simulink library "navlib1"  (Simulink 3.00)
undefined symbols (not defined in the file): Sloc
libraries: navlib1 x10, simulink3 x4
settings Model: LastModifiedBy=Dutchroll

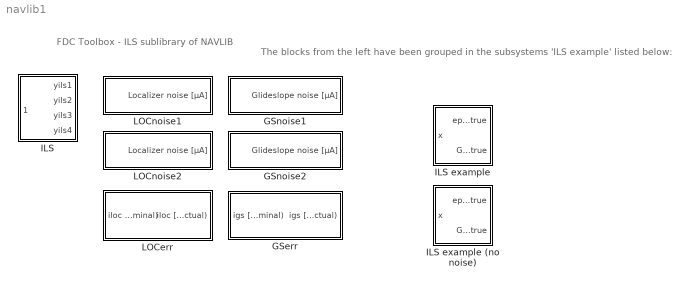
== system navlib1 ==
  note: FDC Toolbox - ILS sublibrary of NAVLIB
  note: The blocks from the left have been
      | grouped in the subsystems
      | 'ILS example' listed below:
  GSerr : Subsystem  mask(GS steady-state errors){cat=2}
      mask prompts: cat "Performance category (1, 2, or 3):"
      mask help: Glideslope steady-state errors
      mask init:
      | gamgs=-abs(@4*pi/180); Sgs=625/abs(gamgs); if cat == 1, D_igs=Sgs*0.075*gamgs; KSgs=1+(@2/100)*0.25; elseif cat == 2, D_igs=Sgs*0.075*gamgs;  KSgs=1+(@2/100)*0.20; else, D_igs=Sgs*0.04*gamgs; KSgs=1+(@2/100)*0.15; end; D_igs=D_igs*@3/100;
      mask Help: eval('browse gserr')
      mask Display: disp('Glideslope steady\nstate errors\nAGARD R-632')
  GSnoise1 : Subsystem  mask(GsNoise1){Lgs=85, sigma_gs=15, V=40}
      mask prompts: Lgs "Scale length Lgs [m]:"; sigma_gs "Standard deviation sigma_gs [µA]:"; V "Approach speed [m/s]:"
      mask help: Glideslope noise (AGARD R-632)
      mask init:
      | K=sigma_gs*sqrt(2*Lgs/V); tau=Lgs/V;
      mask Help: eval('browse gsnoise')
      mask Display: disp('GS noise\nAGARD R-632')
  GSnoise2 : Subsystem
      mask Type: GSNoise NASA-CR2022
      mask Description:
      | Glideslope Noise
      | (NASA-CR2022)
      mask Help: eval('browse gsnoise')
      mask Display: disp('GS noise\nNASA CR-2022')
  ILS : Subsystem  mask(ILS){RWpos=[20000,-100,0]}
      mask prompts: RWpos "Runway heading [deg]:"
      mask help: Approach: ILS
      mask init:
      | psiRW=@1*pi/180; cos_psiRW=cos(psiRW); sin_psiRW=sin(psiRW); xloc=abs(@3); xgs=abs(@4); ygs=-abs(@5); gamgs=-abs(@6)*pi/180; tan_gamgs=tan(gamgs); cos_gamgs=cos(gamgs); Sgs=625/abs(gamgs); if xloc == 0, Sloc = 1; else, Sloc=1.4*xloc; end;
      mask Help: eval('browse ils')
      mask Display: disp('Nominal\nILS\nsignals')
  ILS example : Subsystem
      mask Display: plot(0,0,100,100,[53,23,30,61,53],[45,60,64,49,45],[16,27,32,26],[48,40,43,47],[21,20,24,26,21],[44,55,56,47,44],[20,20,16],[50,50,48],[38,27,26,33],[52,46,48,55],[42,38,27],[50,47,46],[40,44,44,45,45,44,42],[48,44,42,42,44,44,50],[47,45,43],[55,58,58],[54,84,98,90,54],[36,21,56,58,36],[74,68],[34,29],[81,76],[43,38],[87,83],[49,45],[94,89],[57,52],[105,105],[0,0])
  ILS example (no noise) : Subsystem
      mask Display: plot(0,0,100,100,[53,23,30,61,53],[45,60,64,49,45],[16,27,32,26],[48,40,43,47],[21,20,24,26,21],[44,55,56,47,44],[20,20,16],[50,50,48],[38,27,26,33],[52,46,48,55],[42,38,27],[50,47,46],[40,44,44,45,45,44,42],[48,44,42,42,44,44,50],[47,45,43],[55,58,58],[54,84,98,90,54],[36,21,56,58,36],[74,68],[34,29],[81,76],[43,38],[87,83],[49,45],[94,89],[57,52],[105,105],[0,0])
  LOCerr : Subsystem  mask(LOC steady-state errors){cat=2, xloc=2200}
      mask prompts: cat "Performance category (1, 2, or 3):"; xloc "% of max. allowable error in localizer sensitivity:"
      mask help: Localizer steady-state errors
      mask init:
      | Sloc = 1.4*xloc; if cat == 1, D_iloc=Sloc*atan(10.5/xloc); KSloc=1+(@2/100)*0.17; elseif cat == 2, D_iloc=Sloc*atan(7.5/xloc);  KSloc=1+(@2/100)*0.17; else, D_iloc=Sloc*atan(3/xloc); KSloc=1+(@2/100)*0.10; end; D_iloc=D_iloc*@3/100;
      mask Help: eval('browse locerr')
      mask Display: disp('Localizer steady\nstate errors\nAGARD R-632')
  LOCnoise1 : Subsystem  mask(LocNoise1){Lloc=130, sigma_loc=15, V=40}
      mask prompts: Lloc "Scale length Lloc [m]:"; sigma_loc "Standard deviation sigma_loc [µA]:"; V "Approach speed [m/s]:"
      mask help: Localizer noise (AGARD R-632)
      mask init:
      | K=sigma_loc*sqrt(2*Lloc/V); tau=Lloc/V;
      mask Help: eval('browse locnoise')
      mask Display: disp('LOC noise\nAGARD R-632')
  LOCnoise2 : Subsystem
      mask Type: LocNoise 2
      mask Description:
      | Localizer noise
      | (NASA-CR2022)
      mask Help: eval('browse locnoise')
      mask Display: disp('LOC noise\nNASA CR-2022')

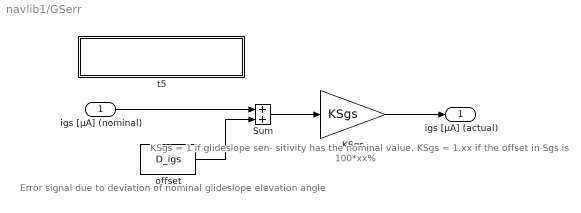
== system navlib1/GSerr ==
  note: KSgs = 1 if glideslope sen-
      | sitivity has the nominal value.
      | KSgs = 1.xx if the offset in
      | Sgs is 100*xx%
  note: Error signal due to deviation
      | of nominal glideslope
      | elevation angle
  igs [µA] (nominal) : Inport  Port=1  PortWidth=-1  SampleTime=-1  DataType=auto
      settings: SignalType=auto
  KSgs : Gain  Gain=KSgs  SaturateOnIntegerOverflow=on
  Sum : Sum  Inputs=++  SaturateOnIntegerOverflow=on
  offset : Constant  Value=D_igs
  t5 : Subsystem
      settings: OpenFcn=browse gserr
      mask Display: disp('Glideslope steady-state errors\nMarc Rauw, April 2003')
  igs [µA] (actual) : Outport  Port=1
  wires:
  offset/1 -> Sum/2
  igs [µA] (nominal)/1 -> Sum/1
  Sum/1 -> KSgs/1
  KSgs/1 -> igs [µA] (actual)/1

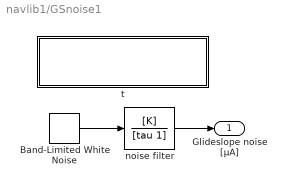
== system navlib1/GSnoise1 ==
  Band-Limited White Noise : simulink3/Sources/Band-Limited White Noise  Cov=[1]  Ts=0.1  seed=[23341]
  noise filter : TransferFcn  Numerator=[K]  Denominator=[tau 1]
  t : Subsystem
      settings: OpenFcn=browse gsnoise
      mask Display: disp('Glideslope noise AGARD R-632\n(constant approach speed)\nMarc Rauw, April 2003')
  Glideslope noise [µA] : Outport  Port=1
  wires:
  Band-Limited White Noise/1 -> noise filter/1
  noise filter/1 -> Glideslope noise [µA]/1

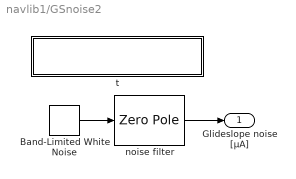
== system navlib1/GSnoise2 ==
  Band-Limited White Noise : simulink3/Sources/Band-Limited White Noise  Cov=[1]  Ts=0.1  seed=[24341]
  noise filter : ZeroPole  Zeros=[]  Poles=[-0.25]  Gain=[3.9875]
  t : Subsystem
      settings: OpenFcn=browse gsnoise
      mask Display: disp('Glideslope noise NASA CR2022\nMarc Rauw, April 2003')
  Glideslope noise [µA] : Outport  Port=1
  wires:
  Band-Limited White Noise/1 -> noise filter/1
  noise filter/1 -> Glideslope noise [µA]/1

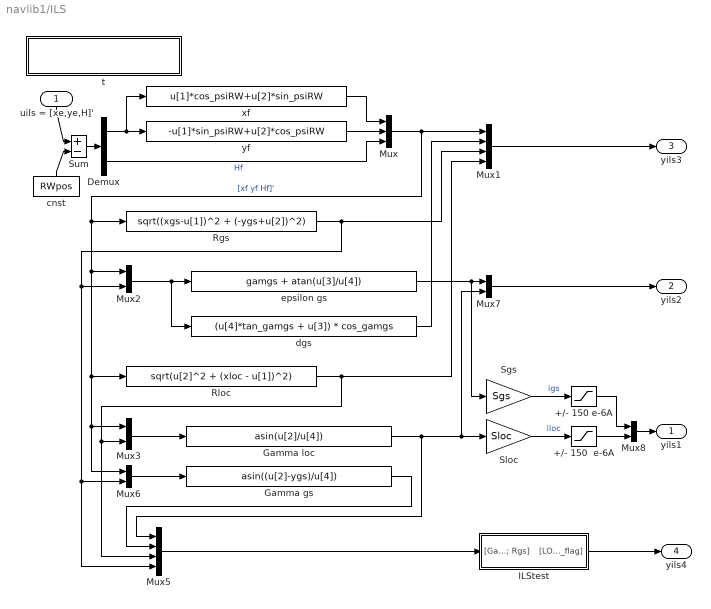
== system navlib1/ILS ==
  uils = [xe,ye,H]' : Inport  Orientation=down  Port=1  PortWidth=-1  SampleTime=-1  DataType=auto
      settings: SignalType=auto
  +/- 150  e-6A : Saturate  UpperLimit=150  LowerLimit=-150
  +/- 150 e-6A : Saturate  UpperLimit=150  LowerLimit=-150
  Demux : Demux  Outputs=[2 1]
  Gamma gs : Fcn  Expr=asin((u[2]-ygs)/u[4])
  Gamma loc : Fcn  Expr=asin(u[2]/u[4])
  ILStest : Subsystem
      mask Type: ILStest
      mask Description: ILS coverage test
      mask Help: eval('browse ilstest')
      mask Display: disp('ILS coverage\ntest (LOC & GS)')
  Mux : Mux  Inputs=3
      settings: DisplayOption=none
  Mux1 : Mux  Inputs=[3 1 1 1]
      settings: DisplayOption=none
  Mux2 : Mux  Inputs=[3 1]
      settings: DisplayOption=none
  Mux3 : Mux  Inputs=[3 1]
      settings: DisplayOption=none
  Mux5 : Mux  Inputs=4
      settings: DisplayOption=none
  Mux6 : Mux  Inputs=[3 1]
      settings: DisplayOption=none
  Mux7 : Mux  Inputs=2
      settings: DisplayOption=none
  Mux8 : Mux  Inputs=2
      settings: DisplayOption=none
  Rgs : Fcn  Expr=sqrt((xgs-u[1])^2 + (-ygs+u[2])^2)
  Rloc : Fcn  Expr=sqrt(u[2]^2 + (xloc - u[1])^2)
  Sgs : Gain  Gain=Sgs  SaturateOnIntegerOverflow=on
  Sloc : Gain  Gain=Sloc  SaturateOnIntegerOverflow=on
  Sum : Sum  Inputs=+-  SaturateOnIntegerOverflow=on
  cnst : Constant  Orientation=up  Value=RWpos
  dgs : Fcn  Expr=(u[4]*tan_gamgs + u[3]) * cos_gamgs
  epsilon gs : Fcn  Expr=gamgs + atan(u[3]/u[4])
  t : Subsystem
      settings: OpenFcn=browse ils
      mask Display: disp('Nominal ILS signals\nM.O. Rauw, February 2004')
  xf : Fcn  Expr=u[1]*cos_psiRW+u[2]*sin_psiRW
  yf : Fcn  Expr=-u[1]*sin_psiRW+u[2]*cos_psiRW
  yils1 : Outport  Port=1
  yils2 : Outport  Port=2
  yils3 : Outport  Port=3
  yils4 : Outport  Port=4
  wires:
  Gamma gs/1 -> Mux5/2
  Mux5/1 -> ILStest/1("[Gamma_loc; Gamma_gs; Rloc; Rgs]")
  ILStest/1("[LOC_flag; GS_flag]") -> yils4/1
  Gamma loc/1 -> Mux5/1, Sloc/1, Mux7/2
  Mux6/1 -> Gamma gs/1
  Mux2/1 -> epsilon gs/1, dgs/1
  Mux1/1 -> yils3/1
  Rloc/1 -> Mux1/4, Mux3/2, Mux5/3
  dgs/1 -> Mux1/2
  Mux3/1 -> Gamma loc/1
  yf/1 -> Mux/2
  xf/1 -> Mux/1
  Sgs/1 -> +/- 150 e-6A/1  "igs"
  Sloc/1 -> +/- 150  e-6A/1  "iloc"
  +/- 150  e-6A/1 -> Mux8/2
  Mux7/1 -> yils2/1
  +/- 150 e-6A/1 -> Mux8/1
  Mux8/1 -> yils1/1
  Rgs/1 -> Mux1/3, Mux2/2, Mux6/2, Mux5/4
  uils = [xe,ye,H]'/1 -> Sum/1
  cnst/1 -> Sum/2
  Demux/2 -> Mux/3  "Hf"
  epsilon gs/1 -> Mux7/1, Sgs/1
  Mux/1 -> Mux2/1, Rloc/1, Mux3/1, Mux6/1, Rgs/1, Mux1/1  "[xf yf Hf]'"
  Sum/1 -> Demux/1
  Demux/1 -> yf/1, xf/1

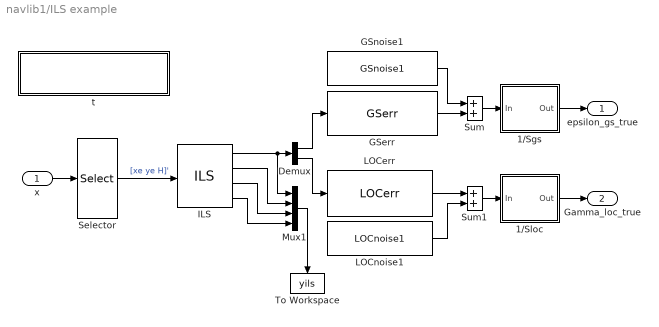
== system navlib1/ILS example ==
  x : Inport  Port=1  PortWidth=-1  SampleTime=-1  DataType=auto
      settings: SignalType=auto
  1/Sgs : Subsystem  mask(1/Sgs){gamgs=-3}
      mask prompts: gamgs "Nominal glideslope angle [deg]:"
      mask help: Multiplication factor 1/Sgs = abs(gamgs)/625, with gamgs the nominal glideslope angle measured in [rad].
      mask init:
      | K = abs(gamgs)*(pi/180)/625;
      mask Help: This block implements a multiplication factor 1/Sgs = abs(gamgs)/625, with gamgs the nominal glideslope angle measured in [rad].
      mask Display: plot([0,100,0,0],[0,50,100,0]);disp('1/Sgs     ');
  1/Sloc : Subsystem  mask(1/Sloc){xloc=2200}
      mask prompts: xloc "Distance from runway threshold to localizer antenna [m]:"
      mask help: Multiplication factor 1/Sloc = 1.40*xloc, with xloc the distance from the runway threshold to the localizer antenna, measured along the runway centerline.
      mask init:
      | K = 1.4*abs(xloc);
      mask Help: This block implements a multiplication factor 1/Sloc = 1.40*xloc, with xloc the distance from the runway threshold to the localizer antenna, measured along the runway centerline.
      mask Display: plot([0,100,0,0],[0,50,100,0]);disp('1/Sloc     ');
  Demux : Demux  Outputs=2
  GSerr : navlib1/GSerr  cat=2  MaskParam2=100  MaskParam3=100  MaskParam4=-3
  GSnoise1 : navlib1/GSnoise1  Lgs=85  sigma_gs=15  V=40
  ILS : navlib1/ILS  RWpos=[20000,-100,0]  MaskParam1=0  MaskParam3=2200  MaskParam4=300  MaskParam5=100  MaskParam6=3
  LOCerr : navlib1/LOCerr  cat=2  xloc=2200  MaskParam2=100  MaskParam3=100
  LOCnoise1 : navlib1/LOCnoise1  Lloc=130  sigma_loc=15  V=40
  Mux1 : Mux  Inputs=[2 2 6 2]
      settings: DisplayOption=none
  Selector : Selector  Elements=[10 11 12]  InputPortWidth=12
  Sum : Sum  Inputs=++  SaturateOnIntegerOverflow=on
  Sum1 : Sum  Inputs=++  SaturateOnIntegerOverflow=on
  To Workspace : ToWorkspace  VariableName=yils  SampleTime=0  SaveFormat=Matrix
      settings: Orientation=down  Buffer=5000
  t : Subsystem
      settings: OpenFcn=browse ilsxmpl
      mask Display: disp('ILS example\nMarc Rauw, January 2005')
  epsilon_gs_true : Outport  Port=1
  Gamma_loc_true : Outport  Port=2
  wires:
  Selector/1 -> ILS/1  "[xe ye H]'"
  Mux1/1 -> To Workspace/1
  Demux/1 -> GSerr/1
  Demux/2 -> LOCerr/1
  ILS/4 -> Mux1/4
  ILS/1 -> Demux/1, Mux1/1
  ILS/3 -> Mux1/3
  ILS/2 -> Mux1/2
  GSerr/1 -> Sum/2
  LOCnoise1/1 -> Sum1/2
  GSnoise1/1 -> Sum/1
  LOCerr/1 -> Sum1/1
  Sum1/1 -> 1/Sloc/1(In)
  Sum/1 -> 1/Sgs/1(In)
  x/1 -> Selector/1
  1/Sgs/1(Out) -> epsilon_gs_true/1
  1/Sloc/1(Out) -> Gamma_loc_true/1

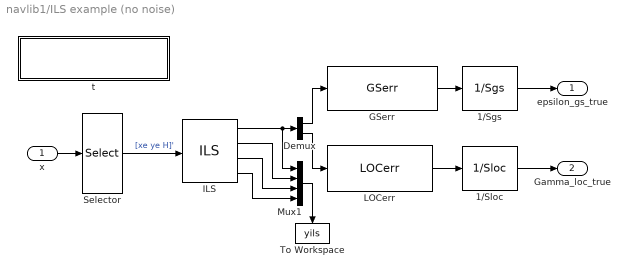
== system navlib1/ILS example (no noise) ==
  x : Inport  Port=1  PortWidth=-1  SampleTime=-1  DataType=auto
      settings: SignalType=auto
  1/Sgs : navlib1/ILS example/1//Sgs  gamgs=-3
  1/Sloc : navlib1/ILS example/1//Sloc  xloc=2200
  Demux : Demux  Outputs=2
  GSerr : navlib1/GSerr  cat=2  MaskParam2=100  MaskParam3=100  MaskParam4=-3
  ILS : navlib1/ILS  RWpos=[20000,-100,0]  MaskParam1=0  MaskParam3=2200  MaskParam4=300  MaskParam5=100  MaskParam6=3
  LOCerr : navlib1/LOCerr  cat=2  xloc=2200  MaskParam2=100  MaskParam3=100
  Mux1 : Mux  Inputs=[2 2 6 2]
      settings: DisplayOption=none
  Selector : Selector  Elements=[10 11 12]  InputPortWidth=12
  To Workspace : ToWorkspace  VariableName=yils  SampleTime=0  SaveFormat=Matrix
      settings: Orientation=down  Buffer=5000
  t : Subsystem
      settings: OpenFcn=browse ilsxmpl
      mask Display: disp('ILS example (no noise)\nMarc Rauw, January 2005')
  epsilon_gs_true : Outport  Port=1
  Gamma_loc_true : Outport  Port=2
  wires:
  Selector/1 -> ILS/1  "[xe ye H]'"
  ILS/2 -> Mux1/2
  ILS/3 -> Mux1/3
  ILS/1 -> Mux1/1, Demux/1
  ILS/4 -> Mux1/4
  Demux/2 -> LOCerr/1
  Demux/1 -> GSerr/1
  Mux1/1 -> To Workspace/1
  x/1 -> Selector/1
  GSerr/1 -> 1/Sgs/1
  1/Sgs/1 -> epsilon_gs_true/1
  LOCerr/1 -> 1/Sloc/1
  1/Sloc/1 -> Gamma_loc_true/1

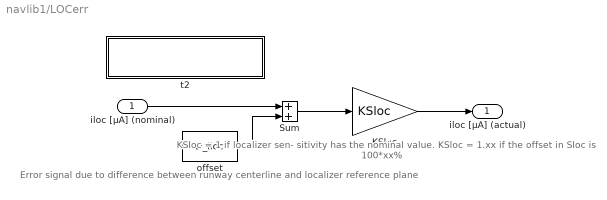
== system navlib1/LOCerr ==
  note: KSloc = 1 if localizer sen-
      | sitivity has the nominal value.
      | KSloc = 1.xx if the offset in
      | Sloc is 100*xx%
  note: Error signal due to difference
      | between runway centerline and
      | localizer reference plane
  iloc [µA] (nominal) : Inport  Port=1  PortWidth=-1  SampleTime=-1  DataType=auto
      settings: SignalType=auto
  KSloc : Gain  Gain=KSloc  SaturateOnIntegerOverflow=on
  Sum : Sum  Inputs=++  SaturateOnIntegerOverflow=on
  offset : Constant  Value=D_iloc
  t2 : Subsystem
      settings: OpenFcn=browse locerr
      mask Display: disp('Localizer steady-state errors\nMarc Rauw, April 2003')
  iloc [µA] (actual) : Outport  Port=1
  wires:
  KSloc/1 -> iloc [µA] (actual)/1
  Sum/1 -> KSloc/1
  iloc [µA] (nominal)/1 -> Sum/1
  offset/1 -> Sum/2

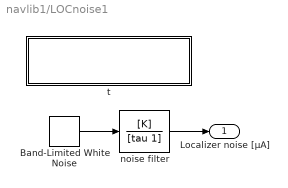
== system navlib1/LOCnoise1 ==
  Band-Limited White Noise : simulink3/Sources/Band-Limited White Noise  Cov=[1]  Ts=0.1  seed=[21341]
  noise filter : TransferFcn  Numerator=[K]  Denominator=[tau 1]
  t : Subsystem
      settings: OpenFcn=browse locnoise
      mask Display: disp('Localizer noise AGARD R-632\n(constant approach speed)\nMarc Rauw, April 2003')
  Localizer noise [µA] : Outport  Port=1
  wires:
  Band-Limited White Noise/1 -> noise filter/1
  noise filter/1 -> Localizer noise [µA]/1

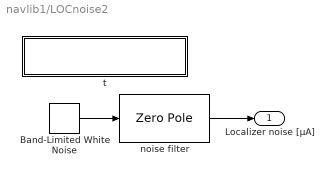
== system navlib1/LOCnoise2 ==
  Band-Limited White Noise : simulink3/Sources/Band-Limited White Noise  Cov=[1]  Ts=0.1  seed=[22341]
  noise filter : ZeroPole  Zeros=[-1.5]  Poles=[-0.35; -10]  Gain=[5]
  t : Subsystem
      settings: OpenFcn=browse locnoise
      mask Display: disp('Localizer noise NASA CR2022\nMarc Rauw, April 2003')
  Localizer noise [µA] : Outport  Port=1
  wires:
  noise filter/1 -> Localizer noise [µA]/1
  Band-Limited White Noise/1 -> noise filter/1

== system navlib1/GSerr/t5 ==
  note: T

== system navlib1/GSnoise1/t ==
  note: T

== system navlib1/GSnoise2/t ==

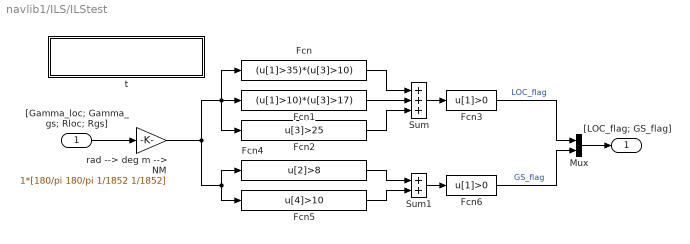
== system navlib1/ILS/ILStest ==
  "[Gamma_loc; Gamma_gs; Rloc; Rgs]" : Inport  Port=1  PortWidth=-1  SampleTime=-1  DataType=auto
      settings: SignalType=auto
  Fcn : Fcn  Expr=(u[1]>35)*(u[3]>10)
  Fcn1 : Fcn  Expr=(u[1]>10)*(u[3]>17)
  Fcn2 : Fcn  Expr=u[3]>25
  Fcn3 : Fcn  Expr=u[1]>0
  Fcn4 : Fcn  Expr=u[2]>8
  Fcn5 : Fcn  Expr=u[4]>10
  Fcn6 : Fcn  Expr=u[1]>0
  Mux : Mux  Inputs=2
      settings: DisplayOption=none
  Sum : Sum  Inputs=+++  SaturateOnIntegerOverflow=on
  Sum1 : Sum  Inputs=++  SaturateOnIntegerOverflow=on
  rad --> deg m --> NM : Gain  Gain=1*[180/pi 180/pi 1/1852 1/1852]  SaturateOnIntegerOverflow=on
  t : Subsystem
      settings: OpenFcn=browse ilstest
      mask Display: disp('ILStest (coverage test)\nM.O. Rauw, February 2004')
  "[LOC_flag; GS_flag]" : Outport  Port=1
  wires:
  "[Gamma_loc; Gamma_gs; Rloc; Rgs]"/1 -> rad --> deg m --> NM/1
  Sum1/1 -> Fcn6/1
  Fcn5/1 -> Sum1/2
  Fcn4/1 -> Sum1/1
  Sum/1 -> Fcn3/1
  Fcn2/1 -> Sum/3
  Fcn1/1 -> Sum/2
  Fcn/1 -> Sum/1
  Mux/1 -> "[LOC_flag; GS_flag]"/1
  Fcn3/1 -> Mux/1  "LOC_flag"
  Fcn6/1 -> Mux/2  "GS_flag"
  rad --> deg m --> NM/1 -> Fcn4/1, Fcn5/1, Fcn1/1, Fcn/1, Fcn2/1

== system navlib1/ILS/t ==

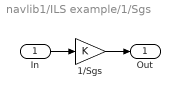
== system navlib1/ILS example/1/Sgs ==
  In : Inport  Port=1  PortWidth=-1  SampleTime=-1  DataType=auto
      settings: SignalType=auto
  1/Sgs : Gain  Gain=K  SaturateOnIntegerOverflow=on
  Out : Outport  Port=1
  wires:
  1/Sgs/1 -> Out/1
  In/1 -> 1/Sgs/1

== system navlib1/ILS example/1/Sloc ==
  In : Inport  Port=1  PortWidth=-1  SampleTime=-1  DataType=auto
      settings: SignalType=auto
  1/Sgs : Gain  Gain=K  SaturateOnIntegerOverflow=on
  Out : Outport  Port=1
  wires:
  In/1 -> 1/Sgs/1
  1/Sgs/1 -> Out/1

== system navlib1/ILS example/t ==

== system navlib1/ILS example (no noise)/t ==

== system navlib1/LOCerr/t2 ==
  note: T

== system navlib1/LOCnoise1/t ==

== system navlib1/LOCnoise2/t ==

== system navlib1/ILS/ILStest/t ==
